simulink model "angle_stab"  (R2015a)
settings: Solver=ode45  StartTime=0.0  StopTime=10  RelTol=1e-3
values from neighbouring files (symbols this model uses):
  alpha_initial = 0    [run.m]
  g = 9.8    [run.m]
  gamma = (k)/(2*m*r)    (= 6.57462195924)    [run.m]
  k = 0.8    [run.m]
  m = 0.078    [run.m]
  W_initial = 0    [run.m]
  x_initial = 0.5    [run.m]
  z_initial = 0.5    [run.m]
undefined symbols (not defined in the file or in its folder): magnitude
settings Model: Creator=Subject 1482  LastModifiedBy=Subject 1482

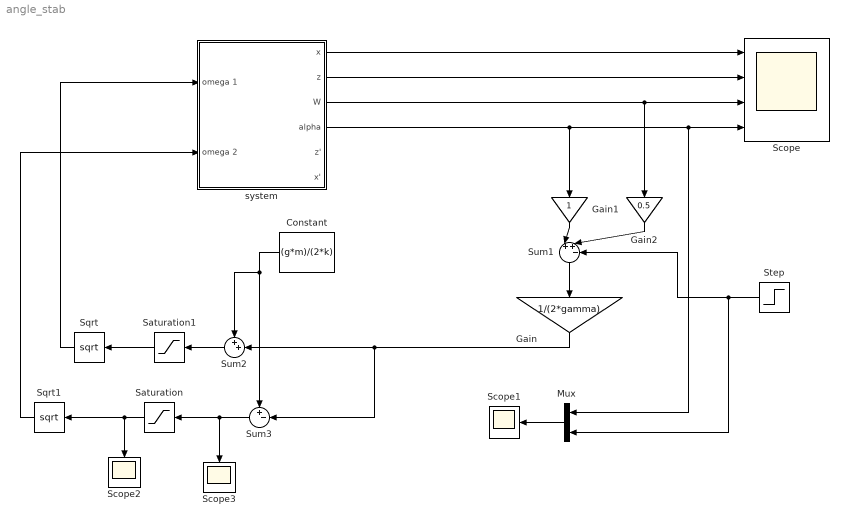
== system angle_stab ==
  Constant : Constant  Value=(g*m)/(2*k)
  Gain : Gain  Gain=1/(2*gamma)
  Gain1 : Gain
  Gain2 : Gain  Gain=0.5
  Mux : Mux  Inputs=2
  Saturation : Saturate  UpperLimit=1000  LowerLimit=0.0001
  Saturation1 : Saturate  UpperLimit=1000  LowerLimit=0.0001
  Scope : Scope  NumInputPorts=4
      settings: TimeRange=10  YMin=0.0405~-405~-160000~-95000  YMax=0.0465~-360~-70000~-45000
  Scope1 : Scope
  Scope2 : Scope
      settings: SaveName=ScopeData2
  Scope3 : Scope
      settings: SaveName=ScopeData3
  Sqrt : Sqrt  SaturateOnIntegerOverflow=on
  Sqrt1 : Sqrt  SaturateOnIntegerOverflow=on
  Step : Step  SampleTime=0
  Sum1 : Sum  Inputs=|++-
  Sum2 : Sum  Inputs=++|
  Sum3 : Sum  Inputs=+-|
  system : Subsystem
  wires:
  system/1(x) -> Scope/1
  system/2(z) -> Scope/2
  system/3(W) -> Gain2/1, Scope/3
  system/4(alpha) -> Mux/1, Scope/4, Gain1/1
  Sum1/1 -> Gain/1
  Constant/1 -> Sum2/1, Sum3/1
  Gain/1 -> Sum3/2, Sum2/2
  Sum2/1 -> Saturation1/1
  Sum3/1 -> Scope3/1, Saturation/1
  Sqrt/1 -> system/1(omega 1)
  Sqrt1/1 -> system/2(omega 2)
  Gain1/1 -> Sum1/1
  Gain2/1 -> Sum1/2
  Step/1 -> Mux/2, Sum1/3
  Mux/1 -> Scope1/1
  Saturation/1 -> Sqrt1/1, Scope2/1
  Saturation1/1 -> Sqrt/1

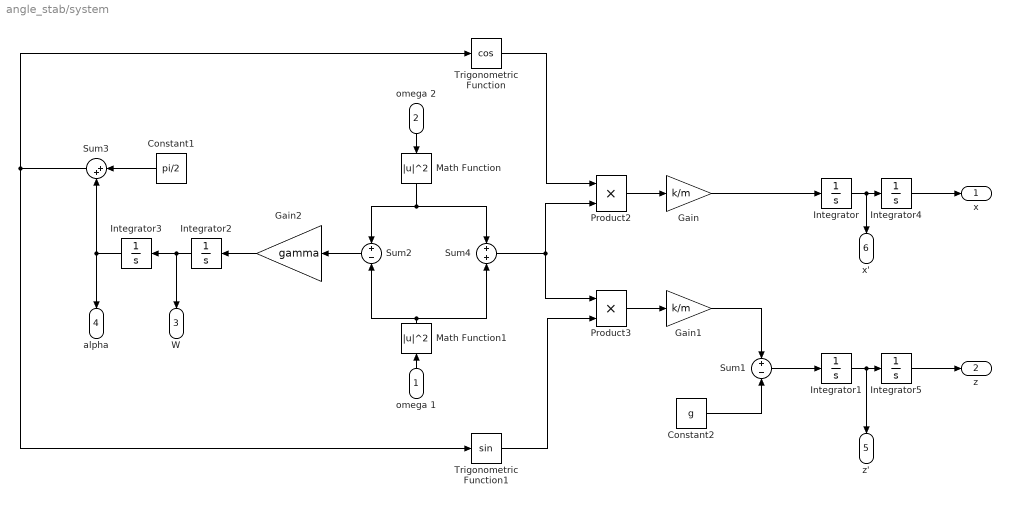
== system angle_stab/system ==
  omega 1 : Inport
  omega 2 : Inport  Port=2
  Constant1 : Constant  Value=pi/2
  Constant2 : Constant  Value=g
  Gain : Gain  Gain=k/m
  Gain1 : Gain  Gain=k/m
  Gain2 : Gain  Gain=gamma
  Integrator : Integrator
  Integrator1 : Integrator
  Integrator2 : Integrator  InitialCondition=W_initial
  Integrator3 : Integrator  InitialCondition=alpha_initial
  Integrator4 : Integrator  InitialCondition=x_initial
  Integrator5 : Integrator  InitialCondition=z_initial
  Math Function : Math  Operator=magnitude^2  SaturateOnIntegerOverflow=on
  Math Function1 : Math  Operator=magnitude^2  SaturateOnIntegerOverflow=on
  Product2 : Product
  Product3 : Product
  Sum1 : Sum  Inputs=+-
  Sum2 : Sum  Inputs=+-
  Sum3 : Sum  Inputs=|++
  Sum4 : Sum
  Trigonometric Function : Trigonometry  Operator=cos
  Trigonometric Function1 : Trigonometry
  x : Outport
  z : Outport  Port=2
  W : Outport  Port=3
  alpha : Outport  Port=4
  z' : Outport  Port=5
  x' : Outport  Port=6
  wires:
  Constant2/1 -> Sum1/2
  Gain1/1 -> Sum1/1
  Sum1/1 -> Integrator1/1
  Product3/1 -> Gain1/1
  Trigonometric Function/1 -> Product2/1
  Gain2/1 -> Integrator2/1
  Integrator3/1 -> Sum3/2, alpha/1
  Trigonometric Function1/1 -> Product3/2
  Product2/1 -> Gain/1
  Gain/1 -> Integrator/1
  Integrator2/1 -> W/1, Integrator3/1
  Constant1/1 -> Sum3/1
  Sum3/1 -> Trigonometric Function1/1, Trigonometric Function/1
  Integrator1/1 -> z'/1, Integrator5/1
  Integrator5/1 -> z/1
  Integrator/1 -> x'/1, Integrator4/1
  Integrator4/1 -> x/1
  omega 2/1 -> Math Function/1
  omega 1/1 -> Math Function1/1
  Sum2/1 -> Gain2/1
  Sum4/1 -> Product3/1, Product2/2
  Math Function1/1 -> Sum2/2, Sum4/2
  Math Function/1 -> Sum4/1, Sum2/1
